simulink model "InportDimensions"  (R2015a)
settings: Solver=FixedStepDiscrete  SolverMode=SingleTasking  StartTime=0.0  StopTime=10.0  RelTol=1e-3
settings Model: CovMetricSettings=dwe  CovHtmlReporting=off  covSaveCumulativeToWorkspaceVar=off  CovSaveSingleToWorkspaceVar=off  CovExternalEMLEnable=on  Creator=hbourbou  LastModifiedBy=hbourbou
settings DataIOCC: LimitDataPoints=off  SaveFormat=Dataset
settings DebuggingCC: SFUnexpectedBacktrackingDiag=error  SFNoUnconditionalDefaultTransitionDiag=error
settings HardwareCC: ProdBitPerPointer=64  ProdLargestAtomicFloat=Float  ProdIntDivRoundTo=Zero  ProdEndianess=LittleEndian  ProdHWDeviceType=Specified
settings ModelReferenceCC: PropagateSignalLabelsOutOfModel=on
settings GRTTargetCC: TargetLangStandard=C99 (ISO)  GeneratePreprocessorConditionals=Use local settings

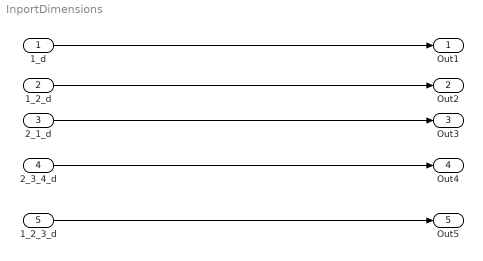
== system InportDimensions ==
  1_d : Inport
  1_2_d : Inport  Port=2  OutDataTypeStr=double  PortDimensions=[1 2]
  2_1_d : Inport  Port=3  PortDimensions=[2 1]
  2_3_4_d : Inport  Port=4  PortDimensions=[2 3 4]
  1_2_3_d : Inport  Port=5  PortDimensions=[1 2 3]
  Out1 : Outport  OutMin=1  OutMax=5
  Out2 : Outport  Port=2
  Out3 : Outport  Port=3
  Out4 : Outport  Port=4
  Out5 : Outport  Port=5
  wires:
  1_d/1 -> Out1/1
  1_2_d/1 -> Out2/1
  2_1_d/1 -> Out3/1
  2_3_4_d/1 -> Out4/1
  1_2_3_d/1 -> Out5/1
